simulink model "ACC_ISO_test_001_cs"  (Simulink 7.6)
settings: Solver=ode5  SolverMode=SingleTasking  StartTime=0.0  StopTime=inf  FixedStep=1/100  RelTol=1e-3
PreLoadFcn:
  | check_NUTS_defined;
  | 
  | assignin('base',['model_closed_' bdroot],false);addpath('../includes_ACC');
InitFcn:
  | PreScanExperimentInitFcn(bdroot)
StopFcn:
  | PreScanExperimentStopFcn(bdroot)
undefined symbols (not defined in the file): DiscIntNeverNeededParam, x_ini_VRML, y_ini_VRML, z_ini_VRML
libraries: simulink x26, PreScanSimulinkLibrary x16, simulink_extras x9, PreScanUsefulBlocks x6, simulink_need_slupdate x1
(part 5 of 9)

== system ACC_ISO_test_001_cs/STATE_Mazda_RX8_1/velRPY ==
  Y : Inport
  Assignment : Assignment  IndexMode=Zero-based  SampleTime=TimeStep  IndexOptions=Starting index (dialog)  Indices=PortIndex  OutputSizes=[1 1]
  Data Store Read : DataStoreRead  DataStoreName=SimCoreActuators  SampleTime=TimeStep
  Data Store Write : DataStoreWrite  DataStoreName=SimCoreActuators
  wires:
  Assignment/1 -> Data Store Write/1
  Data Store Read/1 -> Assignment/1
  Y/1 -> Assignment/2

== system ACC_ISO_test_001_cs/STATE_Sphere_1/Acceleration ==
  Y : Inport
  Assignment : Assignment  IndexMode=Zero-based  SampleTime=TimeStep  IndexOptions=Starting index (dialog)  Indices=PortIndex  OutputSizes=[1 1]
  Data Store Read : DataStoreRead  DataStoreName=SimCoreActuators  SampleTime=TimeStep
  Data Store Write : DataStoreWrite  DataStoreName=SimCoreActuators
  wires:
  Assignment/1 -> Data Store Write/1
  Data Store Read/1 -> Assignment/1
  Y/1 -> Assignment/2

== system ACC_ISO_test_001_cs/STATE_Sphere_1/Position ==
  Y : Inport
  Assignment : Assignment  IndexMode=Zero-based  SampleTime=TimeStep  IndexOptions=Starting index (dialog)  Indices=PortIndex  OutputSizes=[1 1]
  Data Store Read : DataStoreRead  DataStoreName=SimCoreActuators  SampleTime=TimeStep
  Data Store Write : DataStoreWrite  DataStoreName=SimCoreActuators
  wires:
  Y/1 -> Assignment/2
  Data Store Read/1 -> Assignment/1
  Assignment/1 -> Data Store Write/1

== system ACC_ISO_test_001_cs/STATE_Sphere_1/RPY ==
  Y : Inport
  Assignment : Assignment  IndexMode=Zero-based  SampleTime=TimeStep  IndexOptions=Starting index (dialog)  Indices=PortIndex  OutputSizes=[1 1]
  Data Store Read : DataStoreRead  DataStoreName=SimCoreActuators  SampleTime=TimeStep
  Data Store Write : DataStoreWrite  DataStoreName=SimCoreActuators
  wires:
  Assignment/1 -> Data Store Write/1
  Data Store Read/1 -> Assignment/1
  Y/1 -> Assignment/2

== system ACC_ISO_test_001_cs/STATE_Sphere_1/Velocity ==
  Y : Inport
  Assignment : Assignment  IndexMode=Zero-based  SampleTime=TimeStep  IndexOptions=Starting index (dialog)  Indices=PortIndex  OutputSizes=[1 1]
  Data Store Read : DataStoreRead  DataStoreName=SimCoreActuators  SampleTime=TimeStep
  Data Store Write : DataStoreWrite  DataStoreName=SimCoreActuators
  wires:
  Assignment/1 -> Data Store Write/1
  Data Store Read/1 -> Assignment/1
  Y/1 -> Assignment/2

== system ACC_ISO_test_001_cs/STATE_Sphere_1/velRPY ==
  Y : Inport
  Assignment : Assignment  IndexMode=Zero-based  SampleTime=TimeStep  IndexOptions=Starting index (dialog)  Indices=PortIndex  OutputSizes=[1 1]
  Data Store Read : DataStoreRead  DataStoreName=SimCoreActuators  SampleTime=TimeStep
  Data Store Write : DataStoreWrite  DataStoreName=SimCoreActuators
  wires:
  Assignment/1 -> Data Store Write/1
  Data Store Read/1 -> Assignment/1
  Y/1 -> Assignment/2

== system ACC_ISO_test_001_cs/Sphere_1/Dynamics_Empty ==
  note: For state mode 'Dynamic' positions
      | are not taken into account, as they
      | are computed by integrating velocity.
      | Click annotation for Help.
  Ground_{1..9} (9 alike) : Ground
  MuxState : Subsystem  Tag=MuxState  mask{positioningmode=off, TimeStep=1/100}
      mask prompts: positioningmode "Positioning Mode"; TimeStep "Auto Assigned: Time Step [s]"
      settings: DeleteFcn=PreScanBlockDeleteFcn;
  State : Outport  Tag=StateOutport
  wires:
  MuxState/1(state) -> State/1
  Ground_1/1 -> MuxState/1(x [m])
  Ground_2/1 -> MuxState/2(y [m])
  Ground_3/1 -> MuxState/3(z [m])
  Ground_4/1 -> MuxState/4(dx [m/s])
  Ground_5/1 -> MuxState/5(dy [m/s])
  Ground_6/1 -> MuxState/6(dz [m/s])
  Ground_7/1 -> MuxState/7(R [rad])
  Ground_8/1 -> MuxState/8(P [rad])
  Ground_9/1 -> MuxState/9(Y [rad])

== system ACC_ISO_test_001_cs/Sphere_1/SELF_Demux ==
  SELF : Inport
  Demux1 : Demux  Outputs=3
  Demux2 : Demux  Outputs=3
  Demux3 : Demux  Outputs=[3 3 1 1]
  Demux4 : Demux  Outputs=3
  Gain : Gain  Gain=180/pi
  Gain1 : Gain  Gain=180/pi
  Selector : Selector  InputPortWidth=3  IndexOptions=Index vector (dialog)  Indices=[3]  OutputSizes=1
  compas converter : Subsystem
  xyz2GPS : PreScanUsefulBlocks/xyz2GPS  CoordinateCount=1  GPS_base=[0.000000 0.000000 0.000]
  x [m] : Outport
  y [m] : Outport  Port=2
  z [m] : Outport  Port=3
  rotx [deg] : Outport  Port=4
  roty [deg] : Outport  Port=5
  rotz [deg] : Outport  Port=6
  GPS lat [deg] : Outport  Port=7
  GPS long [deg] : Outport  Port=8
  GPS alt [m] : Outport  Port=9
  velocity [m/s] : Outport  Port=10
  heading [deg] : Outport  Port=11
  yaw rate [deg/s] : Outport  Port=12
  wires:
  Demux3/4 -> Gain1/1
  Gain1/1 -> yaw rate [deg/s]/1
  Demux3/3 -> velocity [m/s]/1
  compas converter/1(heading [deg]) -> heading [deg]/1
  xyz2GPS/1 -> Demux4/1
  Demux4/3 -> GPS alt [m]/1
  Demux4/2 -> GPS long [deg]/1
  Demux4/1 -> GPS lat [deg]/1
  Demux3/2 -> Gain/1, Selector/1
  Demux3/1 -> xyz2GPS/1, Demux1/1
  SELF/1 -> Demux3/1
  Demux2/3 -> rotz [deg]/1
  Demux2/2 -> roty [deg]/1
  Demux2/1 -> rotx [deg]/1
  Demux1/3 -> z [m]/1
  Demux1/2 -> y [m]/1
  Demux1/1 -> x [m]/1
  Gain/1 -> Demux2/1
  Selector/1 -> compas converter/1(rotz [rad])

== system ACC_ISO_test_001_cs/VISULightSource_Audi_A8_1/conv_BrakeLightLeft ==
  on_off : Inport
  OffColor : Constant  Value="[51   51   51  255   92    0    0  255  102  102  102  255    0    0    0  255]"
  OnColor : Constant  Value="[51   51   51  255  332   51    0  255  102  102  102  255  583   47    0  255]"
  Switch1 : Switch  Threshold=0.5
  RGBcolor : Outport
  wires:
  OffColor/1 -> Switch1/3  "off"
  OnColor/1 -> Switch1/1  "on"
  on_off/1 -> Switch1/2
  Switch1/1 -> RGBcolor/1

== system ACC_ISO_test_001_cs/VISULightSource_Audi_A8_1/conv_BrakeLightRight ==
  on_off : Inport
  OffColor : Constant  Value="[51   51   51  255   92    0    0  255  102  102  102  255    0    0    0  255]"
  OnColor : Constant  Value="[51   51   51  255  332   51    0  255  102  102  102  255  583   47    0  255]"
  Switch1 : Switch  Threshold=0.5
  RGBcolor : Outport
  wires:
  OffColor/1 -> Switch1/3  "off"
  OnColor/1 -> Switch1/1  "on"
  on_off/1 -> Switch1/2
  Switch1/1 -> RGBcolor/1

== system ACC_ISO_test_001_cs/VISULightSource_Audi_A8_1/conv_FogLightFrontLeft ==
  on_off : Inport
  OffColor : Constant  Value="[51   51   51  255   77   77   77  255  102  102  102  255    0    0    0  255]"
  OnColor : Constant  Value="[51   51   51  255  204  204  204  255  102  102  102  255  510  510  510  255]"
  Switch1 : Switch  Threshold=0.5
  RGBcolor : Outport
  wires:
  OffColor/1 -> Switch1/3  "off"
  OnColor/1 -> Switch1/1  "on"
  on_off/1 -> Switch1/2
  Switch1/1 -> RGBcolor/1

== system ACC_ISO_test_001_cs/VISULightSource_Audi_A8_1/conv_FogLightFrontRight ==
  on_off : Inport
  OffColor : Constant  Value="[51   51   51  255   77   77   77  255  102  102  102  255    0    0    0  255]"
  OnColor : Constant  Value="[51   51   51  255  204  204  204  255  102  102  102  255  510  510  510  255]"
  Switch1 : Switch  Threshold=0.5
  RGBcolor : Outport
  wires:
  OffColor/1 -> Switch1/3  "off"
  OnColor/1 -> Switch1/1  "on"
  on_off/1 -> Switch1/2
  Switch1/1 -> RGBcolor/1

== system ACC_ISO_test_001_cs/VISULightSource_Audi_A8_1/conv_FogLightRearLeft ==
  on_off : Inport
  OffColor : Constant  Value="[51   51   51  255   92    0    0  255  102  102  102  255    0    0    0  255]"
  OnColor : Constant  Value="[51   51   51  255  332   51    0  255  102  102  102  255  583   10    0  255]"
  Switch1 : Switch  Threshold=0.5
  RGBcolor : Outport
  wires:
  OffColor/1 -> Switch1/3  "off"
  OnColor/1 -> Switch1/1  "on"
  on_off/1 -> Switch1/2
  Switch1/1 -> RGBcolor/1

== system ACC_ISO_test_001_cs/VISULightSource_Audi_A8_1/conv_FogLightRearRight ==
  on_off : Inport
  OffColor : Constant  Value="[51   51   51  255   92    0    0  255  102  102  102  255    0    0    0  255]"
  OnColor : Constant  Value="[51   51   51  255  332   51    0  255  102  102  102  255  583   10    0  255]"
  Switch1 : Switch  Threshold=0.5
  RGBcolor : Outport
  wires:
  OffColor/1 -> Switch1/3  "off"
  OnColor/1 -> Switch1/1  "on"
  on_off/1 -> Switch1/2
  Switch1/1 -> RGBcolor/1

== system ACC_ISO_test_001_cs/VISULightSource_Audi_A8_1/conv_IndicatorLightsLeft ==
  on_off : Inport
  OffColor : Constant  Value="[51   51   51  255  138   69    0  255  102  102  102  255    0    0    0  255]"
  OnColor : Constant  Value="[51   51   51  255  255  128    0  255  102  102  102  255  255  191    0  255]"
  Switch1 : Switch  Threshold=0.5
  RGBcolor : Outport
  wires:
  Switch1/1 -> RGBcolor/1
  on_off/1 -> Switch1/2
  OnColor/1 -> Switch1/1  "on"
  OffColor/1 -> Switch1/3  "off"

== system ACC_ISO_test_001_cs/VISULightSource_Audi_A8_1/conv_IndicatorLightsRight ==
  on_off : Inport
  OffColor : Constant  Value="[51   51   51  255  138   69    0  255  102  102  102  255    0    0    0  255]"
  OnColor : Constant  Value="[51   51   51  255  255  128    0  255  102  102  102  255  255  191    0  255]"
  Switch1 : Switch  Threshold=0.5
  RGBcolor : Outport
  wires:
  OffColor/1 -> Switch1/3  "off"
  OnColor/1 -> Switch1/1  "on"
  on_off/1 -> Switch1/2
  Switch1/1 -> RGBcolor/1

== system ACC_ISO_test_001_cs/VISULightSource_Audi_A8_1/conv_MainLightFrontLeft ==
  on_off : Inport
  OffColor : Constant  Value="[26   26   26  255   77   77   77  255  102  102  102  255    0    0    0  255]"
  OnColor : Constant  Value="[51   51   51  255  255  255  255  255  102  102  102  255  683  683  683  255]"
  Switch1 : Switch  Threshold=0.5
  RGBcolor : Outport
  wires:
  OffColor/1 -> Switch1/3  "off"
  OnColor/1 -> Switch1/1  "on"
  on_off/1 -> Switch1/2
  Switch1/1 -> RGBcolor/1

== system ACC_ISO_test_001_cs/VISULightSource_Audi_A8_1/conv_MainLightFrontRight ==
  on_off : Inport
  OffColor : Constant  Value="[26   26   26  255   77   77   77  255  102  102  102  255    0    0    0  255]"
  OnColor : Constant  Value="[51   51   51  255  255  255  255  255  102  102  102  255  683  683  683  255]"
  Switch1 : Switch  Threshold=0.5
  RGBcolor : Outport
  wires:
  OffColor/1 -> Switch1/3  "off"
  OnColor/1 -> Switch1/1  "on"
  on_off/1 -> Switch1/2
  Switch1/1 -> RGBcolor/1

== system ACC_ISO_test_001_cs/VISULightSource_Audi_A8_1/conv_MainLightRearLeft ==
  on_off : Inport
  OffColor : Constant  Value="[51   51   51  255   92    0    0  255  102  102  102  255    0    0    0  255]"
  OnColor : Constant  Value="[51   51   51  255  322   51    0  255  102  102  102  255  255   40    0  255]"
  Switch1 : Switch  Threshold=0.5
  RGBcolor : Outport
  wires:
  OffColor/1 -> Switch1/3  "off"
  OnColor/1 -> Switch1/1  "on"
  on_off/1 -> Switch1/2
  Switch1/1 -> RGBcolor/1

== system ACC_ISO_test_001_cs/VISULightSource_Audi_A8_1/conv_MainLightRearRight ==
  on_off : Inport
  OffColor : Constant  Value="[51   51   51  255   92    0    0  255  102  102  102  255    0    0    0  255]"
  OnColor : Constant  Value="[51   51   51  255  322   51    0  255  102  102  102  255  255   40    0  255]"
  Switch1 : Switch  Threshold=0.5
  RGBcolor : Outport
  wires:
  OffColor/1 -> Switch1/3  "off"
  OnColor/1 -> Switch1/1  "on"
  on_off/1 -> Switch1/2
  Switch1/1 -> RGBcolor/1

== system ACC_ISO_test_001_cs/VISULightSource_Audi_A8_1/visu_BrakeLightLeft_0 ==
  Y : Inport
  Assignment : Assignment  IndexMode=Zero-based  SampleTime=TimeStep  IndexOptions=Starting index (dialog)  Indices=PortIndex  OutputSizes=[1 1]
  Data Store Read : DataStoreRead  DataStoreName=SimCoreActuators  SampleTime=TimeStep
  Data Store Write : DataStoreWrite  DataStoreName=SimCoreActuators
  wires:
  Y/1 -> Assignment/2
  Data Store Read/1 -> Assignment/1
  Assignment/1 -> Data Store Write/1

== system ACC_ISO_test_001_cs/VISULightSource_Audi_A8_1/visu_BrakeLightRight_0 ==
  Y : Inport
  Assignment : Assignment  IndexMode=Zero-based  SampleTime=TimeStep  IndexOptions=Starting index (dialog)  Indices=PortIndex  OutputSizes=[1 1]
  Data Store Read : DataStoreRead  DataStoreName=SimCoreActuators  SampleTime=TimeStep
  Data Store Write : DataStoreWrite  DataStoreName=SimCoreActuators
  wires:
  Y/1 -> Assignment/2
  Data Store Read/1 -> Assignment/1
  Assignment/1 -> Data Store Write/1

== system ACC_ISO_test_001_cs/VISULightSource_Audi_A8_1/visu_FogLightFrontLeft_0 ==
  Y : Inport
  Assignment : Assignment  IndexMode=Zero-based  SampleTime=TimeStep  IndexOptions=Starting index (dialog)  Indices=PortIndex  OutputSizes=[1 1]
  Data Store Read : DataStoreRead  DataStoreName=SimCoreActuators  SampleTime=TimeStep
  Data Store Write : DataStoreWrite  DataStoreName=SimCoreActuators
  wires:
  Y/1 -> Assignment/2
  Data Store Read/1 -> Assignment/1
  Assignment/1 -> Data Store Write/1

== system ACC_ISO_test_001_cs/VISULightSource_Audi_A8_1/visu_FogLightFrontRight_0 ==
  Y : Inport
  Assignment : Assignment  IndexMode=Zero-based  SampleTime=TimeStep  IndexOptions=Starting index (dialog)  Indices=PortIndex  OutputSizes=[1 1]
  Data Store Read : DataStoreRead  DataStoreName=SimCoreActuators  SampleTime=TimeStep
  Data Store Write : DataStoreWrite  DataStoreName=SimCoreActuators
  wires:
  Y/1 -> Assignment/2
  Data Store Read/1 -> Assignment/1
  Assignment/1 -> Data Store Write/1

== system ACC_ISO_test_001_cs/VISULightSource_Audi_A8_1/visu_FogLightRearLeft_0 ==
  Y : Inport
  Assignment : Assignment  IndexMode=Zero-based  SampleTime=TimeStep  IndexOptions=Starting index (dialog)  Indices=PortIndex  OutputSizes=[1 1]
  Data Store Read : DataStoreRead  DataStoreName=SimCoreActuators  SampleTime=TimeStep
  Data Store Write : DataStoreWrite  DataStoreName=SimCoreActuators
  wires:
  Y/1 -> Assignment/2
  Data Store Read/1 -> Assignment/1
  Assignment/1 -> Data Store Write/1

== system ACC_ISO_test_001_cs/VISULightSource_Audi_A8_1/visu_FogLightRearRight_0 ==
  Y : Inport
  Assignment : Assignment  IndexMode=Zero-based  SampleTime=TimeStep  IndexOptions=Starting index (dialog)  Indices=PortIndex  OutputSizes=[1 1]
  Data Store Read : DataStoreRead  DataStoreName=SimCoreActuators  SampleTime=TimeStep
  Data Store Write : DataStoreWrite  DataStoreName=SimCoreActuators
  wires:
  Y/1 -> Assignment/2
  Data Store Read/1 -> Assignment/1
  Assignment/1 -> Data Store Write/1

== system ACC_ISO_test_001_cs/VISULightSource_Audi_A8_1/visu_IndicatorLightsLeft_0 ==
  Y : Inport
  Assignment : Assignment  IndexMode=Zero-based  SampleTime=TimeStep  IndexOptions=Starting index (dialog)  Indices=PortIndex  OutputSizes=[1 1]
  Data Store Read : DataStoreRead  DataStoreName=SimCoreActuators  SampleTime=TimeStep
  Data Store Write : DataStoreWrite  DataStoreName=SimCoreActuators
  wires:
  Assignment/1 -> Data Store Write/1
  Data Store Read/1 -> Assignment/1
  Y/1 -> Assignment/2

== system ACC_ISO_test_001_cs/VISULightSource_Audi_A8_1/visu_IndicatorLightsRight_0 ==
  Y : Inport
  Assignment : Assignment  IndexMode=Zero-based  SampleTime=TimeStep  IndexOptions=Starting index (dialog)  Indices=PortIndex  OutputSizes=[1 1]
  Data Store Read : DataStoreRead  DataStoreName=SimCoreActuators  SampleTime=TimeStep
  Data Store Write : DataStoreWrite  DataStoreName=SimCoreActuators
  wires:
  Y/1 -> Assignment/2
  Data Store Read/1 -> Assignment/1
  Assignment/1 -> Data Store Write/1

== system ACC_ISO_test_001_cs/VISULightSource_Audi_A8_1/visu_MainLightFrontLeft_0 ==
  Y : Inport
  Assignment : Assignment  IndexMode=Zero-based  SampleTime=TimeStep  IndexOptions=Starting index (dialog)  Indices=PortIndex  OutputSizes=[1 1]
  Data Store Read : DataStoreRead  DataStoreName=SimCoreActuators  SampleTime=TimeStep
  Data Store Write : DataStoreWrite  DataStoreName=SimCoreActuators
  wires:
  Y/1 -> Assignment/2
  Data Store Read/1 -> Assignment/1
  Assignment/1 -> Data Store Write/1

== system ACC_ISO_test_001_cs/VISULightSource_Audi_A8_1/visu_MainLightFrontRight_0 ==
  Y : Inport
  Assignment : Assignment  IndexMode=Zero-based  SampleTime=TimeStep  IndexOptions=Starting index (dialog)  Indices=PortIndex  OutputSizes=[1 1]
  Data Store Read : DataStoreRead  DataStoreName=SimCoreActuators  SampleTime=TimeStep
  Data Store Write : DataStoreWrite  DataStoreName=SimCoreActuators
  wires:
  Y/1 -> Assignment/2
  Data Store Read/1 -> Assignment/1
  Assignment/1 -> Data Store Write/1

== system ACC_ISO_test_001_cs/VISULightSource_Audi_A8_1/visu_MainLightRearLeft_0 ==
  Y : Inport
  Assignment : Assignment  IndexMode=Zero-based  SampleTime=TimeStep  IndexOptions=Starting index (dialog)  Indices=PortIndex  OutputSizes=[1 1]
  Data Store Read : DataStoreRead  DataStoreName=SimCoreActuators  SampleTime=TimeStep
  Data Store Write : DataStoreWrite  DataStoreName=SimCoreActuators
  wires:
  Y/1 -> Assignment/2
  Data Store Read/1 -> Assignment/1
  Assignment/1 -> Data Store Write/1

== system ACC_ISO_test_001_cs/VISULightSource_Audi_A8_1/visu_MainLightRearRight_0 ==
  Y : Inport
  Assignment : Assignment  IndexMode=Zero-based  SampleTime=TimeStep  IndexOptions=Starting index (dialog)  Indices=PortIndex  OutputSizes=[1 1]
  Data Store Read : DataStoreRead  DataStoreName=SimCoreActuators  SampleTime=TimeStep
  Data Store Write : DataStoreWrite  DataStoreName=SimCoreActuators
  wires:
  Y/1 -> Assignment/2
  Data Store Read/1 -> Assignment/1
  Assignment/1 -> Data Store Write/1

== system ACC_ISO_test_001_cs/VISULightSource_BMW_X5_1/conv_BrakeLightLeft ==
  on_off : Inport
  OffColor : Constant  Value="[51   51   51  255   92    0    0  255  102  102  102  255    0    0    0  255]"
  OnColor : Constant  Value="[51   51   51  255  332   51    0  255  102  102  102  255  583   47    0  255]"
  Switch1 : Switch  Threshold=0.5
  RGBcolor : Outport
  wires:
  OffColor/1 -> Switch1/3  "off"
  OnColor/1 -> Switch1/1  "on"
  on_off/1 -> Switch1/2
  Switch1/1 -> RGBcolor/1

== system ACC_ISO_test_001_cs/VISULightSource_BMW_X5_1/conv_BrakeLightRight ==
  on_off : Inport
  OffColor : Constant  Value="[51   51   51  255   92    0    0  255  102  102  102  255    0    0    0  255]"
  OnColor : Constant  Value="[51   51   51  255  332   51    0  255  102  102  102  255  583   47    0  255]"
  Switch1 : Switch  Threshold=0.5
  RGBcolor : Outport
  wires:
  OffColor/1 -> Switch1/3  "off"
  OnColor/1 -> Switch1/1  "on"
  on_off/1 -> Switch1/2
  Switch1/1 -> RGBcolor/1

== system ACC_ISO_test_001_cs/VISULightSource_BMW_X5_1/conv_FogLightFrontLeft ==
  on_off : Inport
  OffColor : Constant  Value="[51   51   51  255   77   77   77  255  102  102  102  255    0    0    0  255]"
  OnColor : Constant  Value="[51   51   51  255  204  204  204  255  102  102  102  255  510  510  510  255]"
  Switch1 : Switch  Threshold=0.5
  RGBcolor : Outport
  wires:
  OffColor/1 -> Switch1/3  "off"
  OnColor/1 -> Switch1/1  "on"
  on_off/1 -> Switch1/2
  Switch1/1 -> RGBcolor/1

== system ACC_ISO_test_001_cs/VISULightSource_BMW_X5_1/conv_FogLightFrontRight ==
  on_off : Inport
  OffColor : Constant  Value="[51   51   51  255   77   77   77  255  102  102  102  255    0    0    0  255]"
  OnColor : Constant  Value="[51   51   51  255  204  204  204  255  102  102  102  255  510  510  510  255]"
  Switch1 : Switch  Threshold=0.5
  RGBcolor : Outport
  wires:
  OffColor/1 -> Switch1/3  "off"
  OnColor/1 -> Switch1/1  "on"
  on_off/1 -> Switch1/2
  Switch1/1 -> RGBcolor/1

== system ACC_ISO_test_001_cs/VISULightSource_BMW_X5_1/conv_FogLightRearLeft ==
  on_off : Inport
  OffColor : Constant  Value="[51   51   51  255   92    0    0  255  102  102  102  255    0    0    0  255]"
  OnColor : Constant  Value="[51   51   51  255  332   51    0  255  102  102  102  255  583   10    0  255]"
  Switch1 : Switch  Threshold=0.5
  RGBcolor : Outport
  wires:
  OffColor/1 -> Switch1/3  "off"
  OnColor/1 -> Switch1/1  "on"
  on_off/1 -> Switch1/2
  Switch1/1 -> RGBcolor/1

== system ACC_ISO_test_001_cs/VISULightSource_BMW_X5_1/conv_FogLightRearRight ==
  on_off : Inport
  OffColor : Constant  Value="[51   51   51  255   92    0    0  255  102  102  102  255    0    0    0  255]"
  OnColor : Constant  Value="[51   51   51  255  332   51    0  255  102  102  102  255  583   10    0  255]"
  Switch1 : Switch  Threshold=0.5
  RGBcolor : Outport
  wires:
  OffColor/1 -> Switch1/3  "off"
  OnColor/1 -> Switch1/1  "on"
  on_off/1 -> Switch1/2
  Switch1/1 -> RGBcolor/1

== system ACC_ISO_test_001_cs/VISULightSource_BMW_X5_1/conv_IndicatorLightsLeft ==
  on_off : Inport
  OffColor : Constant  Value="[51   51   51  255  138   69    0  255  102  102  102  255    0    0    0  255]"
  OnColor : Constant  Value="[51   51   51  255  255  128    0  255  102  102  102  255  255  191    0  255]"
  Switch1 : Switch  Threshold=0.5
  RGBcolor : Outport
  wires:
  Switch1/1 -> RGBcolor/1
  on_off/1 -> Switch1/2
  OnColor/1 -> Switch1/1  "on"
  OffColor/1 -> Switch1/3  "off"

== system ACC_ISO_test_001_cs/VISULightSource_BMW_X5_1/conv_IndicatorLightsRight ==
  on_off : Inport
  OffColor : Constant  Value="[51   51   51  255  138   69    0  255  102  102  102  255    0    0    0  255]"
  OnColor : Constant  Value="[51   51   51  255  255  128    0  255  102  102  102  255  255  191    0  255]"
  Switch1 : Switch  Threshold=0.5
  RGBcolor : Outport
  wires:
  OffColor/1 -> Switch1/3  "off"
  OnColor/1 -> Switch1/1  "on"
  on_off/1 -> Switch1/2
  Switch1/1 -> RGBcolor/1

== system ACC_ISO_test_001_cs/VISULightSource_BMW_X5_1/conv_MainLightFrontLeft ==
  on_off : Inport
  OffColor : Constant  Value="[26   26   26  255   77   77   77  255  102  102  102  255    0    0    0  255]"
  OnColor : Constant  Value="[51   51   51  255  255  255  255  255  102  102  102  255  683  683  683  255]"
  Switch1 : Switch  Threshold=0.5
  RGBcolor : Outport
  wires:
  OffColor/1 -> Switch1/3  "off"
  OnColor/1 -> Switch1/1  "on"
  on_off/1 -> Switch1/2
  Switch1/1 -> RGBcolor/1

== system ACC_ISO_test_001_cs/VISULightSource_BMW_X5_1/conv_MainLightFrontRight ==
  on_off : Inport
  OffColor : Constant  Value="[26   26   26  255   77   77   77  255  102  102  102  255    0    0    0  255]"
  OnColor : Constant  Value="[51   51   51  255  255  255  255  255  102  102  102  255  683  683  683  255]"
  Switch1 : Switch  Threshold=0.5
  RGBcolor : Outport
  wires:
  OffColor/1 -> Switch1/3  "off"
  OnColor/1 -> Switch1/1  "on"
  on_off/1 -> Switch1/2
  Switch1/1 -> RGBcolor/1

== system ACC_ISO_test_001_cs/VISULightSource_BMW_X5_1/conv_MainLightRearLeft ==
  on_off : Inport
  OffColor : Constant  Value="[51   51   51  255   92    0    0  255  102  102  102  255    0    0    0  255]"
  OnColor : Constant  Value="[51   51   51  255  322   51    0  255  102  102  102  255  255   40    0  255]"
  Switch1 : Switch  Threshold=0.5
  RGBcolor : Outport
  wires:
  OffColor/1 -> Switch1/3  "off"
  OnColor/1 -> Switch1/1  "on"
  on_off/1 -> Switch1/2
  Switch1/1 -> RGBcolor/1

== system ACC_ISO_test_001_cs/VISULightSource_BMW_X5_1/conv_MainLightRearRight ==
  on_off : Inport
  OffColor : Constant  Value="[51   51   51  255   92    0    0  255  102  102  102  255    0    0    0  255]"
  OnColor : Constant  Value="[51   51   51  255  322   51    0  255  102  102  102  255  255   40    0  255]"
  Switch1 : Switch  Threshold=0.5
  RGBcolor : Outport
  wires:
  OffColor/1 -> Switch1/3  "off"
  OnColor/1 -> Switch1/1  "on"
  on_off/1 -> Switch1/2
  Switch1/1 -> RGBcolor/1

== system ACC_ISO_test_001_cs/VISULightSource_BMW_X5_1/visu_BrakeLightLeft_0 ==
  Y : Inport
  Assignment : Assignment  IndexMode=Zero-based  SampleTime=TimeStep  IndexOptions=Starting index (dialog)  Indices=PortIndex  OutputSizes=[1 1]
  Data Store Read : DataStoreRead  DataStoreName=SimCoreActuators  SampleTime=TimeStep
  Data Store Write : DataStoreWrite  DataStoreName=SimCoreActuators
  wires:
  Y/1 -> Assignment/2
  Data Store Read/1 -> Assignment/1
  Assignment/1 -> Data Store Write/1

== system ACC_ISO_test_001_cs/VISULightSource_BMW_X5_1/visu_BrakeLightRight_0 ==
  Y : Inport
  Assignment : Assignment  IndexMode=Zero-based  SampleTime=TimeStep  IndexOptions=Starting index (dialog)  Indices=PortIndex  OutputSizes=[1 1]
  Data Store Read : DataStoreRead  DataStoreName=SimCoreActuators  SampleTime=TimeStep
  Data Store Write : DataStoreWrite  DataStoreName=SimCoreActuators
  wires:
  Y/1 -> Assignment/2
  Data Store Read/1 -> Assignment/1
  Assignment/1 -> Data Store Write/1

== system ACC_ISO_test_001_cs/VISULightSource_BMW_X5_1/visu_FogLightFrontLeft_0 ==
  Y : Inport
  Assignment : Assignment  IndexMode=Zero-based  SampleTime=TimeStep  IndexOptions=Starting index (dialog)  Indices=PortIndex  OutputSizes=[1 1]
  Data Store Read : DataStoreRead  DataStoreName=SimCoreActuators  SampleTime=TimeStep
  Data Store Write : DataStoreWrite  DataStoreName=SimCoreActuators
  wires:
  Y/1 -> Assignment/2
  Data Store Read/1 -> Assignment/1
  Assignment/1 -> Data Store Write/1

== system ACC_ISO_test_001_cs/VISULightSource_BMW_X5_1/visu_FogLightFrontRight_0 ==
  Y : Inport
  Assignment : Assignment  IndexMode=Zero-based  SampleTime=TimeStep  IndexOptions=Starting index (dialog)  Indices=PortIndex  OutputSizes=[1 1]
  Data Store Read : DataStoreRead  DataStoreName=SimCoreActuators  SampleTime=TimeStep
  Data Store Write : DataStoreWrite  DataStoreName=SimCoreActuators
  wires:
  Y/1 -> Assignment/2
  Data Store Read/1 -> Assignment/1
  Assignment/1 -> Data Store Write/1

== system ACC_ISO_test_001_cs/VISULightSource_BMW_X5_1/visu_FogLightRearLeft_0 ==
  Y : Inport
  Assignment : Assignment  IndexMode=Zero-based  SampleTime=TimeStep  IndexOptions=Starting index (dialog)  Indices=PortIndex  OutputSizes=[1 1]
  Data Store Read : DataStoreRead  DataStoreName=SimCoreActuators  SampleTime=TimeStep
  Data Store Write : DataStoreWrite  DataStoreName=SimCoreActuators
  wires:
  Y/1 -> Assignment/2
  Data Store Read/1 -> Assignment/1
  Assignment/1 -> Data Store Write/1

== system ACC_ISO_test_001_cs/VISULightSource_BMW_X5_1/visu_FogLightRearRight_0 ==
  Y : Inport
  Assignment : Assignment  IndexMode=Zero-based  SampleTime=TimeStep  IndexOptions=Starting index (dialog)  Indices=PortIndex  OutputSizes=[1 1]
  Data Store Read : DataStoreRead  DataStoreName=SimCoreActuators  SampleTime=TimeStep
  Data Store Write : DataStoreWrite  DataStoreName=SimCoreActuators
  wires:
  Y/1 -> Assignment/2
  Data Store Read/1 -> Assignment/1
  Assignment/1 -> Data Store Write/1

== system ACC_ISO_test_001_cs/VISULightSource_BMW_X5_1/visu_IndicatorLightsLeft_0 ==
  Y : Inport
  Assignment : Assignment  IndexMode=Zero-based  SampleTime=TimeStep  IndexOptions=Starting index (dialog)  Indices=PortIndex  OutputSizes=[1 1]
  Data Store Read : DataStoreRead  DataStoreName=SimCoreActuators  SampleTime=TimeStep
  Data Store Write : DataStoreWrite  DataStoreName=SimCoreActuators
  wires:
  Assignment/1 -> Data Store Write/1
  Data Store Read/1 -> Assignment/1
  Y/1 -> Assignment/2

== system ACC_ISO_test_001_cs/VISULightSource_BMW_X5_1/visu_IndicatorLightsRight_0 ==
  Y : Inport
  Assignment : Assignment  IndexMode=Zero-based  SampleTime=TimeStep  IndexOptions=Starting index (dialog)  Indices=PortIndex  OutputSizes=[1 1]
  Data Store Read : DataStoreRead  DataStoreName=SimCoreActuators  SampleTime=TimeStep
  Data Store Write : DataStoreWrite  DataStoreName=SimCoreActuators
  wires:
  Y/1 -> Assignment/2
  Data Store Read/1 -> Assignment/1
  Assignment/1 -> Data Store Write/1

== system ACC_ISO_test_001_cs/VISULightSource_BMW_X5_1/visu_MainLightFrontLeft_0 ==
  Y : Inport
  Assignment : Assignment  IndexMode=Zero-based  SampleTime=TimeStep  IndexOptions=Starting index (dialog)  Indices=PortIndex  OutputSizes=[1 1]
  Data Store Read : DataStoreRead  DataStoreName=SimCoreActuators  SampleTime=TimeStep
  Data Store Write : DataStoreWrite  DataStoreName=SimCoreActuators
  wires:
  Y/1 -> Assignment/2
  Data Store Read/1 -> Assignment/1
  Assignment/1 -> Data Store Write/1

== system ACC_ISO_test_001_cs/VISULightSource_BMW_X5_1/visu_MainLightFrontRight_0 ==
  Y : Inport
  Assignment : Assignment  IndexMode=Zero-based  SampleTime=TimeStep  IndexOptions=Starting index (dialog)  Indices=PortIndex  OutputSizes=[1 1]
  Data Store Read : DataStoreRead  DataStoreName=SimCoreActuators  SampleTime=TimeStep
  Data Store Write : DataStoreWrite  DataStoreName=SimCoreActuators
  wires:
  Y/1 -> Assignment/2
  Data Store Read/1 -> Assignment/1
  Assignment/1 -> Data Store Write/1

== system ACC_ISO_test_001_cs/VISULightSource_BMW_X5_1/visu_MainLightRearLeft_0 ==
  Y : Inport
  Assignment : Assignment  IndexMode=Zero-based  SampleTime=TimeStep  IndexOptions=Starting index (dialog)  Indices=PortIndex  OutputSizes=[1 1]
  Data Store Read : DataStoreRead  DataStoreName=SimCoreActuators  SampleTime=TimeStep
  Data Store Write : DataStoreWrite  DataStoreName=SimCoreActuators
  wires:
  Y/1 -> Assignment/2
  Data Store Read/1 -> Assignment/1
  Assignment/1 -> Data Store Write/1

== system ACC_ISO_test_001_cs/VISULightSource_BMW_X5_1/visu_MainLightRearRight_0 ==
  Y : Inport
  Assignment : Assignment  IndexMode=Zero-based  SampleTime=TimeStep  IndexOptions=Starting index (dialog)  Indices=PortIndex  OutputSizes=[1 1]
  Data Store Read : DataStoreRead  DataStoreName=SimCoreActuators  SampleTime=TimeStep
  Data Store Write : DataStoreWrite  DataStoreName=SimCoreActuators
  wires:
  Y/1 -> Assignment/2
  Data Store Read/1 -> Assignment/1
  Assignment/1 -> Data Store Write/1

== system ACC_ISO_test_001_cs/VISULightSource_Mazda_RX8_1/conv_BrakeLightLeft ==
  on_off : Inport
  OffColor : Constant  Value="[51   51   51  255   92    0    0  255  102  102  102  255    0    0    0  255]"
  OnColor : Constant  Value="[51   51   51  255  332   51    0  255  102  102  102  255  583   47    0  255]"
  Switch1 : Switch  Threshold=0.5
  RGBcolor : Outport
  wires:
  OffColor/1 -> Switch1/3  "off"
  OnColor/1 -> Switch1/1  "on"
  on_off/1 -> Switch1/2
  Switch1/1 -> RGBcolor/1

== system ACC_ISO_test_001_cs/VISULightSource_Mazda_RX8_1/conv_BrakeLightMiddle ==
  on_off : Inport
  OffColor : Constant  Value="[51   51   51  255   92    0    0  255  102  102  102  255    0    0    0  255]"
  OnColor : Constant  Value="[51   51   51  255  332   51    0  255  102  102  102  255  583   47    0  255]"
  Switch1 : Switch  Threshold=0.5
  RGBcolor : Outport
  wires:
  OffColor/1 -> Switch1/3  "off"
  OnColor/1 -> Switch1/1  "on"
  on_off/1 -> Switch1/2
  Switch1/1 -> RGBcolor/1

== system ACC_ISO_test_001_cs/VISULightSource_Mazda_RX8_1/conv_BrakeLightRight ==
  on_off : Inport
  OffColor : Constant  Value="[51   51   51  255   92    0    0  255  102  102  102  255    0    0    0  255]"
  OnColor : Constant  Value="[51   51   51  255  332   51    0  255  102  102  102  255  583   47    0  255]"
  Switch1 : Switch  Threshold=0.5
  RGBcolor : Outport
  wires:
  OffColor/1 -> Switch1/3  "off"
  OnColor/1 -> Switch1/1  "on"
  on_off/1 -> Switch1/2
  Switch1/1 -> RGBcolor/1

== system ACC_ISO_test_001_cs/VISULightSource_Mazda_RX8_1/conv_FogLightFrontLeft ==
  on_off : Inport
  OffColor : Constant  Value="[51   51   51  255   77   77   77  255  102  102  102  255    0    0    0  255]"
  OnColor : Constant  Value="[51   51   51  255  204  204  204  255  102  102  102  255  510  510  510  255]"
  Switch1 : Switch  Threshold=0.5
  RGBcolor : Outport
  wires:
  OffColor/1 -> Switch1/3  "off"
  OnColor/1 -> Switch1/1  "on"
  on_off/1 -> Switch1/2
  Switch1/1 -> RGBcolor/1

== system ACC_ISO_test_001_cs/VISULightSource_Mazda_RX8_1/conv_FogLightFrontRight ==
  on_off : Inport
  OffColor : Constant  Value="[51   51   51  255   77   77   77  255  102  102  102  255    0    0    0  255]"
  OnColor : Constant  Value="[51   51   51  255  204  204  204  255  102  102  102  255  510  510  510  255]"
  Switch1 : Switch  Threshold=0.5
  RGBcolor : Outport
  wires:
  OffColor/1 -> Switch1/3  "off"
  OnColor/1 -> Switch1/1  "on"
  on_off/1 -> Switch1/2
  Switch1/1 -> RGBcolor/1

== system ACC_ISO_test_001_cs/VISULightSource_Mazda_RX8_1/conv_FogLightRearLeft ==
  on_off : Inport
  OffColor : Constant  Value="[51   51   51  255   92    0    0  255  102  102  102  255    0    0    0  255]"
  OnColor : Constant  Value="[51   51   51  255  332   51    0  255  102  102  102  255  583   10    0  255]"
  Switch1 : Switch  Threshold=0.5
  RGBcolor : Outport
  wires:
  OffColor/1 -> Switch1/3  "off"
  OnColor/1 -> Switch1/1  "on"
  on_off/1 -> Switch1/2
  Switch1/1 -> RGBcolor/1

== system ACC_ISO_test_001_cs/VISULightSource_Mazda_RX8_1/conv_FogLightRearRight ==
  on_off : Inport
  OffColor : Constant  Value="[51   51   51  255   92    0    0  255  102  102  102  255    0    0    0  255]"
  OnColor : Constant  Value="[51   51   51  255  332   51    0  255  102  102  102  255  583   10    0  255]"
  Switch1 : Switch  Threshold=0.5
  RGBcolor : Outport
  wires:
  OffColor/1 -> Switch1/3  "off"
  OnColor/1 -> Switch1/1  "on"
  on_off/1 -> Switch1/2
  Switch1/1 -> RGBcolor/1

== system ACC_ISO_test_001_cs/VISULightSource_Mazda_RX8_1/conv_IndicatorLightsLeft ==
  on_off : Inport
  OffColor : Constant  Value="[51   51   51  255  138   69    0  255  102  102  102  255    0    0    0  255]"
  OnColor : Constant  Value="[51   51   51  255  255  128    0  255  102  102  102  255  255  191    0  255]"
  Switch1 : Switch  Threshold=0.5
  RGBcolor : Outport
  wires:
  Switch1/1 -> RGBcolor/1
  on_off/1 -> Switch1/2
  OnColor/1 -> Switch1/1  "on"
  OffColor/1 -> Switch1/3  "off"

== system ACC_ISO_test_001_cs/VISULightSource_Mazda_RX8_1/conv_IndicatorLightsRight ==
  on_off : Inport
  OffColor : Constant  Value="[51   51   51  255  138   69    0  255  102  102  102  255    0    0    0  255]"
  OnColor : Constant  Value="[51   51   51  255  255  128    0  255  102  102  102  255  255  191    0  255]"
  Switch1 : Switch  Threshold=0.5
  RGBcolor : Outport
  wires:
  OffColor/1 -> Switch1/3  "off"
  OnColor/1 -> Switch1/1  "on"
  on_off/1 -> Switch1/2
  Switch1/1 -> RGBcolor/1

== system ACC_ISO_test_001_cs/VISULightSource_Mazda_RX8_1/conv_MainLightFrontLeft ==
  on_off : Inport
  OffColor : Constant  Value="[26   26   26  255   77   77   77  255  102  102  102  255    0    0    0  255]"
  OnColor : Constant  Value="[51   51   51  255  255  255  255  255  102  102  102  255  683  683  683  255]"
  Switch1 : Switch  Threshold=0.5
  RGBcolor : Outport
  wires:
  OffColor/1 -> Switch1/3  "off"
  OnColor/1 -> Switch1/1  "on"
  on_off/1 -> Switch1/2
  Switch1/1 -> RGBcolor/1

== system ACC_ISO_test_001_cs/VISULightSource_Mazda_RX8_1/conv_MainLightFrontRight ==
  on_off : Inport
  OffColor : Constant  Value="[26   26   26  255   77   77   77  255  102  102  102  255    0    0    0  255]"
  OnColor : Constant  Value="[51   51   51  255  255  255  255  255  102  102  102  255  683  683  683  255]"
  Switch1 : Switch  Threshold=0.5
  RGBcolor : Outport
  wires:
  OffColor/1 -> Switch1/3  "off"
  OnColor/1 -> Switch1/1  "on"
  on_off/1 -> Switch1/2
  Switch1/1 -> RGBcolor/1

== system ACC_ISO_test_001_cs/VISULightSource_Mazda_RX8_1/conv_MainLightRearLeft ==
  on_off : Inport
  OffColor : Constant  Value="[51   51   51  255   92    0    0  255  102  102  102  255    0    0    0  255]"
  OnColor : Constant  Value="[51   51   51  255  322   51    0  255  102  102  102  255  255   40    0  255]"
  Switch1 : Switch  Threshold=0.5
  RGBcolor : Outport
  wires:
  OffColor/1 -> Switch1/3  "off"
  OnColor/1 -> Switch1/1  "on"
  on_off/1 -> Switch1/2
  Switch1/1 -> RGBcolor/1

== system ACC_ISO_test_001_cs/VISULightSource_Mazda_RX8_1/conv_MainLightRearRight ==
  on_off : Inport
  OffColor : Constant  Value="[51   51   51  255   92    0    0  255  102  102  102  255    0    0    0  255]"
  OnColor : Constant  Value="[51   51   51  255  322   51    0  255  102  102  102  255  255   40    0  255]"
  Switch1 : Switch  Threshold=0.5
  RGBcolor : Outport
  wires:
  OffColor/1 -> Switch1/3  "off"
  OnColor/1 -> Switch1/1  "on"
  on_off/1 -> Switch1/2
  Switch1/1 -> RGBcolor/1

== system ACC_ISO_test_001_cs/VISULightSource_Mazda_RX8_1/visu_BrakeLightLeft_0 ==
  Y : Inport
  Assignment : Assignment  IndexMode=Zero-based  SampleTime=TimeStep  IndexOptions=Starting index (dialog)  Indices=PortIndex  OutputSizes=[1 1]
  Data Store Read : DataStoreRead  DataStoreName=SimCoreActuators  SampleTime=TimeStep
  Data Store Write : DataStoreWrite  DataStoreName=SimCoreActuators
  wires:
  Y/1 -> Assignment/2
  Data Store Read/1 -> Assignment/1
  Assignment/1 -> Data Store Write/1

== system ACC_ISO_test_001_cs/VISULightSource_Mazda_RX8_1/visu_BrakeLightMiddle_0 ==
  Y : Inport
  Assignment : Assignment  IndexMode=Zero-based  SampleTime=TimeStep  IndexOptions=Starting index (dialog)  Indices=PortIndex  OutputSizes=[1 1]
  Data Store Read : DataStoreRead  DataStoreName=SimCoreActuators  SampleTime=TimeStep
  Data Store Write : DataStoreWrite  DataStoreName=SimCoreActuators
  wires:
  Y/1 -> Assignment/2
  Data Store Read/1 -> Assignment/1
  Assignment/1 -> Data Store Write/1

== system ACC_ISO_test_001_cs/VISULightSource_Mazda_RX8_1/visu_BrakeLightRight_0 ==
  Y : Inport
  Assignment : Assignment  IndexMode=Zero-based  SampleTime=TimeStep  IndexOptions=Starting index (dialog)  Indices=PortIndex  OutputSizes=[1 1]
  Data Store Read : DataStoreRead  DataStoreName=SimCoreActuators  SampleTime=TimeStep
  Data Store Write : DataStoreWrite  DataStoreName=SimCoreActuators
  wires:
  Y/1 -> Assignment/2
  Data Store Read/1 -> Assignment/1
  Assignment/1 -> Data Store Write/1

== system ACC_ISO_test_001_cs/VISULightSource_Mazda_RX8_1/visu_FogLightFrontLeft_0 ==
  Y : Inport
  Assignment : Assignment  IndexMode=Zero-based  SampleTime=TimeStep  IndexOptions=Starting index (dialog)  Indices=PortIndex  OutputSizes=[1 1]
  Data Store Read : DataStoreRead  DataStoreName=SimCoreActuators  SampleTime=TimeStep
  Data Store Write : DataStoreWrite  DataStoreName=SimCoreActuators
  wires:
  Y/1 -> Assignment/2
  Data Store Read/1 -> Assignment/1
  Assignment/1 -> Data Store Write/1

== system ACC_ISO_test_001_cs/VISULightSource_Mazda_RX8_1/visu_FogLightFrontRight_0 ==
  Y : Inport
  Assignment : Assignment  IndexMode=Zero-based  SampleTime=TimeStep  IndexOptions=Starting index (dialog)  Indices=PortIndex  OutputSizes=[1 1]
  Data Store Read : DataStoreRead  DataStoreName=SimCoreActuators  SampleTime=TimeStep
  Data Store Write : DataStoreWrite  DataStoreName=SimCoreActuators
  wires:
  Y/1 -> Assignment/2
  Data Store Read/1 -> Assignment/1
  Assignment/1 -> Data Store Write/1

== system ACC_ISO_test_001_cs/VISULightSource_Mazda_RX8_1/visu_FogLightRearLeft_0 ==
  Y : Inport
  Assignment : Assignment  IndexMode=Zero-based  SampleTime=TimeStep  IndexOptions=Starting index (dialog)  Indices=PortIndex  OutputSizes=[1 1]
  Data Store Read : DataStoreRead  DataStoreName=SimCoreActuators  SampleTime=TimeStep
  Data Store Write : DataStoreWrite  DataStoreName=SimCoreActuators
  wires:
  Y/1 -> Assignment/2
  Data Store Read/1 -> Assignment/1
  Assignment/1 -> Data Store Write/1

== system ACC_ISO_test_001_cs/VISULightSource_Mazda_RX8_1/visu_FogLightRearRight_0 ==
  Y : Inport
  Assignment : Assignment  IndexMode=Zero-based  SampleTime=TimeStep  IndexOptions=Starting index (dialog)  Indices=PortIndex  OutputSizes=[1 1]
  Data Store Read : DataStoreRead  DataStoreName=SimCoreActuators  SampleTime=TimeStep
  Data Store Write : DataStoreWrite  DataStoreName=SimCoreActuators
  wires:
  Y/1 -> Assignment/2
  Data Store Read/1 -> Assignment/1
  Assignment/1 -> Data Store Write/1

== system ACC_ISO_test_001_cs/VISULightSource_Mazda_RX8_1/visu_IndicatorLightsLeft_0 ==
  Y : Inport
  Assignment : Assignment  IndexMode=Zero-based  SampleTime=TimeStep  IndexOptions=Starting index (dialog)  Indices=PortIndex  OutputSizes=[1 1]
  Data Store Read : DataStoreRead  DataStoreName=SimCoreActuators  SampleTime=TimeStep
  Data Store Write : DataStoreWrite  DataStoreName=SimCoreActuators
  wires:
  Assignment/1 -> Data Store Write/1
  Data Store Read/1 -> Assignment/1
  Y/1 -> Assignment/2

== system ACC_ISO_test_001_cs/VISULightSource_Mazda_RX8_1/visu_IndicatorLightsRight_0 ==
  Y : Inport
  Assignment : Assignment  IndexMode=Zero-based  SampleTime=TimeStep  IndexOptions=Starting index (dialog)  Indices=PortIndex  OutputSizes=[1 1]
  Data Store Read : DataStoreRead  DataStoreName=SimCoreActuators  SampleTime=TimeStep
  Data Store Write : DataStoreWrite  DataStoreName=SimCoreActuators
  wires:
  Y/1 -> Assignment/2
  Data Store Read/1 -> Assignment/1
  Assignment/1 -> Data Store Write/1

== system ACC_ISO_test_001_cs/VISULightSource_Mazda_RX8_1/visu_MainLightFrontLeft_0 ==
  Y : Inport
  Assignment : Assignment  IndexMode=Zero-based  SampleTime=TimeStep  IndexOptions=Starting index (dialog)  Indices=PortIndex  OutputSizes=[1 1]
  Data Store Read : DataStoreRead  DataStoreName=SimCoreActuators  SampleTime=TimeStep
  Data Store Write : DataStoreWrite  DataStoreName=SimCoreActuators
  wires:
  Y/1 -> Assignment/2
  Data Store Read/1 -> Assignment/1
  Assignment/1 -> Data Store Write/1

== system ACC_ISO_test_001_cs/VISULightSource_Mazda_RX8_1/visu_MainLightFrontRight_0 ==
  Y : Inport
  Assignment : Assignment  IndexMode=Zero-based  SampleTime=TimeStep  IndexOptions=Starting index (dialog)  Indices=PortIndex  OutputSizes=[1 1]
  Data Store Read : DataStoreRead  DataStoreName=SimCoreActuators  SampleTime=TimeStep
  Data Store Write : DataStoreWrite  DataStoreName=SimCoreActuators
  wires:
  Y/1 -> Assignment/2
  Data Store Read/1 -> Assignment/1
  Assignment/1 -> Data Store Write/1

== system ACC_ISO_test_001_cs/VISULightSource_Mazda_RX8_1/visu_MainLightRearLeft_0 ==
  Y : Inport
  Assignment : Assignment  IndexMode=Zero-based  SampleTime=TimeStep  IndexOptions=Starting index (dialog)  Indices=PortIndex  OutputSizes=[1 1]
  Data Store Read : DataStoreRead  DataStoreName=SimCoreActuators  SampleTime=TimeStep
  Data Store Write : DataStoreWrite  DataStoreName=SimCoreActuators
  wires:
  Y/1 -> Assignment/2
  Data Store Read/1 -> Assignment/1
  Assignment/1 -> Data Store Write/1

== system ACC_ISO_test_001_cs/VISULightSource_Mazda_RX8_1/visu_MainLightRearRight_0 ==
  Y : Inport
  Assignment : Assignment  IndexMode=Zero-based  SampleTime=TimeStep  IndexOptions=Starting index (dialog)  Indices=PortIndex  OutputSizes=[1 1]
  Data Store Read : DataStoreRead  DataStoreName=SimCoreActuators  SampleTime=TimeStep
  Data Store Write : DataStoreWrite  DataStoreName=SimCoreActuators
  wires:
  Y/1 -> Assignment/2
  Data Store Read/1 -> Assignment/1
  Assignment/1 -> Data Store Write/1

== system ACC_ISO_test_001_cs/VISUSteer_Audi_A8_1/conv_SteeringColumn ==
  angle [deg] : Inport
  Constant13 : Constant  Value=[0 1 0]
  Mux8 : Mux  Inputs=2
  deg2rad : Gain  Gain=pi/180
  QuaternionVisu [rad] : Outport
  wires:
  deg2rad/1 -> Mux8/2
  Constant13/1 -> Mux8/1
  Mux8/1 -> QuaternionVisu [rad]/1
  angle [deg]/1 -> deg2rad/1

== system ACC_ISO_test_001_cs/VISUSteer_Audi_A8_1/conv_SteeringWheel ==
  angle [deg] : Inport
  Constant13 : Constant  Value=[-1 0 0]
  Mux8 : Mux  Inputs=2
  deg2rad : Gain  Gain=pi/180
  QuaternionVisu [rad] : Outport
  wires:
  deg2rad/1 -> Mux8/2
  Constant13/1 -> Mux8/1
  Mux8/1 -> QuaternionVisu [rad]/1
  angle [deg]/1 -> deg2rad/1

== system ACC_ISO_test_001_cs/VISUSteer_Audi_A8_1/visu_SteeringColumn ==
  Y : Inport
  Assignment : Assignment  IndexMode=Zero-based  SampleTime=TimeStep  IndexOptions=Starting index (dialog)  Indices=PortIndex  OutputSizes=[1 1]
  Data Store Read : DataStoreRead  DataStoreName=SimCoreActuators  SampleTime=TimeStep
  Data Store Write : DataStoreWrite  DataStoreName=SimCoreActuators
  wires:
  Assignment/1 -> Data Store Write/1
  Data Store Read/1 -> Assignment/1
  Y/1 -> Assignment/2

== system ACC_ISO_test_001_cs/VISUSteer_Audi_A8_1/visu_SteeringWheel ==
  Y : Inport
  Assignment : Assignment  IndexMode=Zero-based  SampleTime=TimeStep  IndexOptions=Starting index (dialog)  Indices=PortIndex  OutputSizes=[1 1]
  Data Store Read : DataStoreRead  DataStoreName=SimCoreActuators  SampleTime=TimeStep
  Data Store Write : DataStoreWrite  DataStoreName=SimCoreActuators
  wires:
  Assignment/1 -> Data Store Write/1
  Data Store Read/1 -> Assignment/1
  Y/1 -> Assignment/2

== system ACC_ISO_test_001_cs/VISUSteer_BMW_X5_1/conv_SteeringColumn ==
  angle [deg] : Inport
  Constant13 : Constant  Value=[0 1 0]
  Mux8 : Mux  Inputs=2
  deg2rad : Gain  Gain=pi/180
  QuaternionVisu [rad] : Outport
  wires:
  deg2rad/1 -> Mux8/2
  Constant13/1 -> Mux8/1
  Mux8/1 -> QuaternionVisu [rad]/1
  angle [deg]/1 -> deg2rad/1

== system ACC_ISO_test_001_cs/VISUSteer_BMW_X5_1/conv_SteeringWheel ==
  angle [deg] : Inport
  Constant13 : Constant  Value=[-1 0 0]
  Mux8 : Mux  Inputs=2
  deg2rad : Gain  Gain=pi/180
  QuaternionVisu [rad] : Outport
  wires:
  deg2rad/1 -> Mux8/2
  Constant13/1 -> Mux8/1
  Mux8/1 -> QuaternionVisu [rad]/1
  angle [deg]/1 -> deg2rad/1

== system ACC_ISO_test_001_cs/VISUSteer_BMW_X5_1/visu_SteeringColumn ==
  Y : Inport
  Assignment : Assignment  IndexMode=Zero-based  SampleTime=TimeStep  IndexOptions=Starting index (dialog)  Indices=PortIndex  OutputSizes=[1 1]
  Data Store Read : DataStoreRead  DataStoreName=SimCoreActuators  SampleTime=TimeStep
  Data Store Write : DataStoreWrite  DataStoreName=SimCoreActuators
  wires:
  Assignment/1 -> Data Store Write/1
  Data Store Read/1 -> Assignment/1
  Y/1 -> Assignment/2

== system ACC_ISO_test_001_cs/VISUSteer_BMW_X5_1/visu_SteeringWheel ==
  Y : Inport
  Assignment : Assignment  IndexMode=Zero-based  SampleTime=TimeStep  IndexOptions=Starting index (dialog)  Indices=PortIndex  OutputSizes=[1 1]
  Data Store Read : DataStoreRead  DataStoreName=SimCoreActuators  SampleTime=TimeStep
  Data Store Write : DataStoreWrite  DataStoreName=SimCoreActuators
  wires:
  Assignment/1 -> Data Store Write/1
  Data Store Read/1 -> Assignment/1
  Y/1 -> Assignment/2

== system ACC_ISO_test_001_cs/VISUSteer_Mazda_RX8_1/conv_SteeringColumn ==
  angle [deg] : Inport
  Constant13 : Constant  Value=[0 1 0]
  Mux8 : Mux  Inputs=2
  deg2rad : Gain  Gain=pi/180
  QuaternionVisu [rad] : Outport
  wires:
  deg2rad/1 -> Mux8/2
  Constant13/1 -> Mux8/1
  Mux8/1 -> QuaternionVisu [rad]/1
  angle [deg]/1 -> deg2rad/1

== system ACC_ISO_test_001_cs/VISUSteer_Mazda_RX8_1/conv_SteeringWheel ==
  angle [deg] : Inport
  Constant13 : Constant  Value=[-1 0 0]
  Mux8 : Mux  Inputs=2
  deg2rad : Gain  Gain=pi/180
  QuaternionVisu [rad] : Outport
  wires:
  deg2rad/1 -> Mux8/2
  Constant13/1 -> Mux8/1
  Mux8/1 -> QuaternionVisu [rad]/1
  angle [deg]/1 -> deg2rad/1

== system ACC_ISO_test_001_cs/VISUSteer_Mazda_RX8_1/visu_SteeringColumn ==
  Y : Inport
  Assignment : Assignment  IndexMode=Zero-based  SampleTime=TimeStep  IndexOptions=Starting index (dialog)  Indices=PortIndex  OutputSizes=[1 1]
  Data Store Read : DataStoreRead  DataStoreName=SimCoreActuators  SampleTime=TimeStep
  Data Store Write : DataStoreWrite  DataStoreName=SimCoreActuators
  wires:
  Assignment/1 -> Data Store Write/1
  Data Store Read/1 -> Assignment/1
  Y/1 -> Assignment/2

== system ACC_ISO_test_001_cs/VISUSteer_Mazda_RX8_1/visu_SteeringWheel ==
  Y : Inport
  Assignment : Assignment  IndexMode=Zero-based  SampleTime=TimeStep  IndexOptions=Starting index (dialog)  Indices=PortIndex  OutputSizes=[1 1]
  Data Store Read : DataStoreRead  DataStoreName=SimCoreActuators  SampleTime=TimeStep
  Data Store Write : DataStoreWrite  DataStoreName=SimCoreActuators
  wires:
  Assignment/1 -> Data Store Write/1
  Data Store Read/1 -> Assignment/1
  Y/1 -> Assignment/2
